simulink model "ECE551_ex1"  (R2018a)
settings: Solver=ode23tb  StartTime=0.0  StopTime=50  RelTol=1e-3
settings Model: Creator=clarke6  LastModifiedBy=clarke6

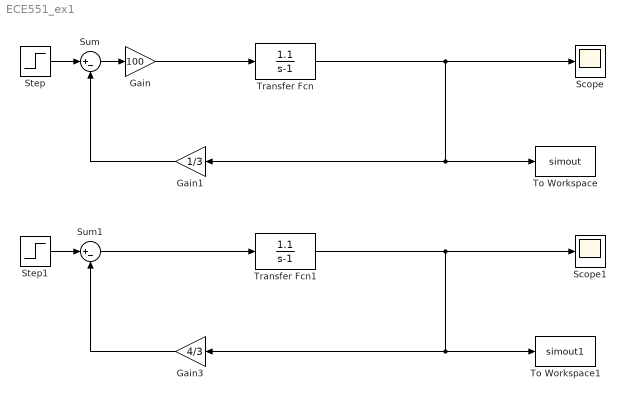
== system ECE551_ex1 ==
  Gain : Gain  Gain=100
  Gain1 : Gain  Gain=1/3
  Gain3 : Gain  Gain=4/3
  Scope : Scope
  Scope1 : Scope
  Step : Step  SampleTime=0
  Step1 : Step  SampleTime=0
  Sum : Sum  Inputs=|+-
  Sum1 : Sum  Inputs=|+-
  To Workspace : ToWorkspace  VariableName=simout  SaveFormat=Timeseries  SampleTime=-1
  To Workspace1 : ToWorkspace  VariableName=simout1  SaveFormat=Timeseries  SampleTime=-1
  Transfer Fcn : TransferFcn  Numerator=[1.1]  Denominator=[1 -1]
  Transfer Fcn1 : TransferFcn  Numerator=[1.1]  Denominator=[1 -1]
  wires:
  Sum/1 -> Gain/1
  Step/1 -> Sum/1
  Gain/1 -> Transfer Fcn/1
  Transfer Fcn/1 -> To Workspace/1, Gain1/1, Scope/1
  Gain1/1 -> Sum/2
  Sum1/1 -> Transfer Fcn1/1
  Step1/1 -> Sum1/1
  Gain3/1 -> Sum1/2
  Transfer Fcn1/1 -> To Workspace1/1, Gain3/1, Scope1/1
